simulink model "DvrSimKeybdGD_cs_old"  (R2016a)
settings: Solver=ode5  SolverMode=SingleTasking  StartTime=0.0  StopTime=inf  FixedStep=1/1000  RelTol=1e-3
PreLoadFcn:
  | mbxruntime.callbacks.PreLoadFcn(bdroot);
PostLoadFcn:
  | mbxruntime.callbacks.PostLoadFcn(bdroot);
InitFcn:
  | mbxruntime.callbacks.InitFcn(bdroot);
StartFcn:
  | mbxruntime.callbacks.StartFcn(bdroot);
StopFcn:
  | mbxruntime.callbacks.StopFcn(bdroot);
model workspace (MAT data in the model file):
  mbox_table : struct (value not decoded)
  model_closed = 0
  sim_status = 0
undefined symbols (not defined in the file or in its folder): BMotor1, BMotor2, BrkDelayTime, DControlB, Delay1, Delay2, DiscIntNeverNeededParam, IControlB, JMotor1, JMotor2, PControlB, PreScanCarSimLoadFcn, ratioGearF, ratioGearR, TorqDelayTime, Tstep
undefined symbols (not defined in the file): SteeringColumn, SteeringWheel, WheelL0, WheelL1, WheelR0, WheelR1
libraries: PreScanSimulinkLibrary x35, simulink_extras x26, simulink x26, MyLib x3, Solver_SF x2, pil_lib x1, PreScanUsefulBlocks x1
(part 9 of 12)

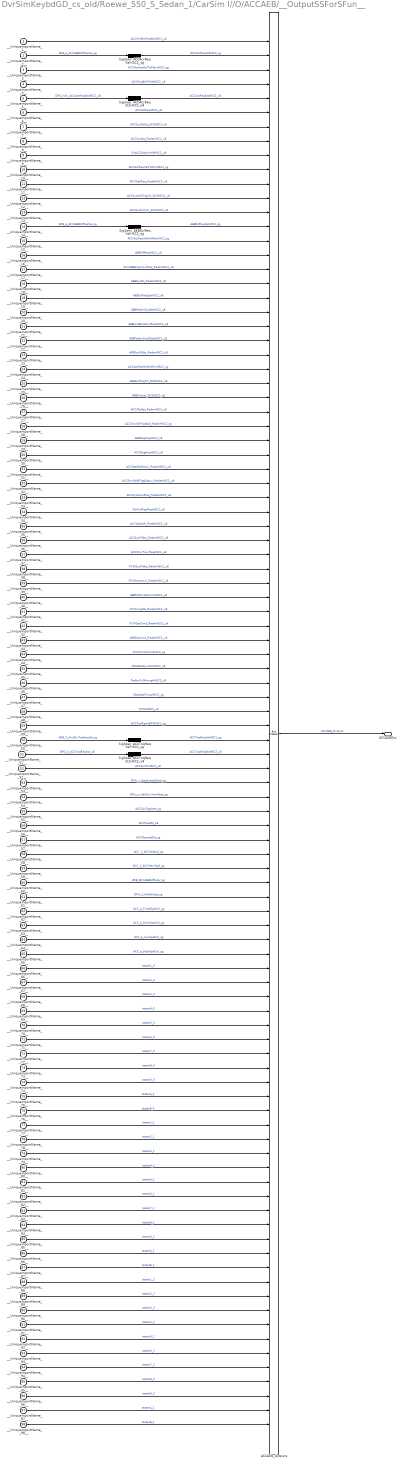
== system DvrSimKeybdGD_cs_old/Roewe_550_S_Sedan_1/CarSim I//O/ACCAEB/__OutputSSForSFun__ ==
  __UniqueInportName__1__ : Inport
  __UniqueInportName__2__ : Inport  Port=2
  __UniqueInportName__3__ : Inport  Port=3
  __UniqueInportName__4__ : Inport  Port=4
  __UniqueInportName__5__ : Inport  Port=5
  __UniqueInportName__6__ : Inport  Port=6
  __UniqueInportName__7__ : Inport  Port=7
  __UniqueInportName__8__ : Inport  Port=8
  __UniqueInportName__9__ : Inport  Port=9
  __UniqueInportName__10__ : Inport  Port=10
  __UniqueInportName__11__ : Inport  Port=11
  __UniqueInportName__12__ : Inport  Port=12
  __UniqueInportName__13__ : Inport  Port=13
  __UniqueInportName__14__ : Inport  Port=14
  __UniqueInportName__15__ : Inport  Port=15
  __UniqueInportName__16__ : Inport  Port=16
  __UniqueInportName__17__ : Inport  Port=17
  __UniqueInportName__18__ : Inport  Port=18
  __UniqueInportName__19__ : Inport  Port=19
  __UniqueInportName__20__ : Inport  Port=20
  __UniqueInportName__21__ : Inport  Port=21
  __UniqueInportName__22__ : Inport  Port=22
  __UniqueInportName__23__ : Inport  Port=23
  __UniqueInportName__24__ : Inport  Port=24
  __UniqueInportName__25__ : Inport  Port=25
  __UniqueInportName__26__ : Inport  Port=26
  __UniqueInportName__27__ : Inport  Port=27
  __UniqueInportName__28__ : Inport  Port=28
  __UniqueInportName__29__ : Inport  Port=29
  __UniqueInportName__30__ : Inport  Port=30
  __UniqueInportName__31__ : Inport  Port=31
  __UniqueInportName__32__ : Inport  Port=32
  __UniqueInportName__33__ : Inport  Port=33
  __UniqueInportName__34__ : Inport  Port=34
  __UniqueInportName__35__ : Inport  Port=35
  __UniqueInportName__36__ : Inport  Port=36
  __UniqueInportName__37__ : Inport  Port=37
  __UniqueInportName__38__ : Inport  Port=38
  __UniqueInportName__39__ : Inport  Port=39
  __UniqueInportName__40__ : Inport  Port=40
  __UniqueInportName__41__ : Inport  Port=41
  __UniqueInportName__42__ : Inport  Port=42
  __UniqueInportName__43__ : Inport  Port=43
  __UniqueInportName__44__ : Inport  Port=44
  __UniqueInportName__45__ : Inport  Port=45
  __UniqueInportName__46__ : Inport  Port=46
  __UniqueInportName__47__ : Inport  Port=47
  __UniqueInportName__48__ : Inport  Port=48
  __UniqueInportName__49__ : Inport  Port=49
  __UniqueInportName__50__ : Inport  Port=50
  __UniqueInportName__51__ : Inport  Port=51
  __UniqueInportName__52__ : Inport  Port=52
  __UniqueInportName__53__ : Inport  Port=53
  __UniqueInportName__54__ : Inport  Port=54
  __UniqueInportName__55__ : Inport  Port=55
  __UniqueInportName__56__ : Inport  Port=56
  __UniqueInportName__57__ : Inport  Port=57
  __UniqueInportName__58__ : Inport  Port=58
  __UniqueInportName__59__ : Inport  Port=59
  __UniqueInportName__60__ : Inport  Port=60
  __UniqueInportName__61__ : Inport  Port=61
  __UniqueInportName__62__ : Inport  Port=62
  __UniqueInportName__63__ : Inport  Port=63
  __UniqueInportName__64__ : Inport  Port=64
  __UniqueInportName__65__ : Inport  Port=65
  __UniqueInportName__66__ : Inport  Port=66
  __UniqueInportName__67__ : Inport  Port=67
  __UniqueInportName__68__ : Inport  Port=68
  __UniqueInportName__69__ : Inport  Port=69
  __UniqueInportName__70__ : Inport  Port=70
  __UniqueInportName__71__ : Inport  Port=71
  __UniqueInportName__72__ : Inport  Port=72
  __UniqueInportName__73__ : Inport  Port=73
  __UniqueInportName__74__ : Inport  Port=74
  __UniqueInportName__75__ : Inport  Port=75
  __UniqueInportName__76__ : Inport  Port=76
  __UniqueInportName__77__ : Inport  Port=77
  __UniqueInportName__78__ : Inport  Port=78
  __UniqueInportName__79__ : Inport  Port=79
  __UniqueInportName__80__ : Inport  Port=80
  __UniqueInportName__81__ : Inport  Port=81
  __UniqueInportName__82__ : Inport  Port=82
  __UniqueInportName__83__ : Inport  Port=83
  __UniqueInportName__84__ : Inport  Port=84
  __UniqueInportName__85__ : Inport  Port=85
  __UniqueInportName__86__ : Inport  Port=86
  __UniqueInportName__87__ : Inport  Port=87
  __UniqueInportName__88__ : Inport  Port=88
  __UniqueInportName__89__ : Inport  Port=89
  __UniqueInportName__90__ : Inport  Port=90
  __UniqueInportName__91__ : Inport  Port=91
  __UniqueInportName__92__ : Inport  Port=92
  __UniqueInportName__93__ : Inport  Port=93
  __UniqueInportName__94__ : Inport  Port=94
  __UniqueInportName__95__ : Inport  Port=95
  __UniqueInportName__96__ : Inport  Port=96
  __UniqueInportName__97__ : Inport  Port=97
  __UniqueInportName__98__ : Inport  Port=98
  ACCAEB_Outputs : BusCreator  Inputs=98
  SigSpec_ACCAccReqStsHSC2_u8 : Demux  Outputs=1
  SigSpec_ACCAccReqValHSC2_sg : Demux  Outputs=1
  SigSpec_ACCToqReqStsHSC2_u8 : Demux  Outputs=1
  SigSpec_ACCToqReqValHSC2_sg : Demux  Outputs=1
  SigSpec_AEBDclReqValHSC2_sg : Demux  Outputs=1
  ACCAEBOut : Outport
  wires:
  __UniqueInportName__2__/1 -> SigSpec_ACCAccReqValHSC2_sg/1  "ARB_a_ACCAEBDclReqVal_sg"
  __UniqueInportName__5__/1 -> SigSpec_ACCAccReqStsHSC2_u8/1  "DPO_indx_ACCAccReqStsHSC2_u8"
  __UniqueInportName__14__/1 -> SigSpec_AEBDclReqValHSC2_sg/1  "ARB_a_ACCAEBDclReqVal_sg"
  __UniqueInportName__50__/1 -> SigSpec_ACCToqReqValHSC2_sg/1  "ARB_T_SmtDrvToqReqVal_sg"
  __UniqueInportName__51__/1 -> SigSpec_ACCToqReqStsHSC2_u8/1  "DPO_is_ACCToqReqSts_u8"
  __UniqueInportName__1__/1 -> ACCAEB_Outputs/1  "ACCMinBrkReqStsHSC2_u8"
  SigSpec_ACCAccReqValHSC2_sg/1 -> ACCAEB_Outputs/2  "ACCAccReqValHSC2_sg"
  __UniqueInportName__3__/1 -> ACCAEB_Outputs/3  "ACCAccReqValTolMaxHSC2_sg"
  __UniqueInportName__4__/1 -> ACCAEB_Outputs/4  "ACCReqBrkPrfrdHSC2_u8"
  SigSpec_ACCAccReqStsHSC2_u8/1 -> ACCAEB_Outputs/5  "ACCAccReqStsHSC2_u8"
  __UniqueInportName__6__/1 -> ACCAEB_Outputs/6  "ACCGoReqHSC2_u8"
  __UniqueInportName__7__/1 -> ACCAEB_Outputs/7  "ACCSysFltSts_SCSHSC2_u8"
  __UniqueInportName__8__/1 -> ACCAEB_Outputs/8  "ACCSysSts_RadarHSC2_u8"
  __UniqueInportName__9__/1 -> ACCAEB_Outputs/9  "ChACCShtdwnMdHSC2_u8"
  __UniqueInportName__10__/1 -> ACCAEB_Outputs/10  "ACCAccReqValTolMinHSC2_sg"
  __UniqueInportName__11__/1 -> ACCAEB_Outputs/11  "ACCSdslReq_RadarHSC2_u8"
  __UniqueInportName__12__/1 -> ACCAEB_Outputs/12  "ACCSysAlvRlngCtr_SCSHSC2_u8"
  __UniqueInportName__13__/1 -> ACCAEB_Outputs/13  "ACCSysChksm_SCSHSC2_u8"
  SigSpec_AEBDclReqValHSC2_sg/1 -> ACCAEB_Outputs/14  "AEBDclReqValHSC2_sg"
  __UniqueInportName__15__/1 -> ACCAEB_Outputs/15  "ACCAccReqValGrdMaxHSC2_sg"
  __UniqueInportName__16__/1 -> ACCAEB_Outputs/16  "AEBPrflReqHSC2_u8"
  __UniqueInportName__17__/1 -> ACCAEB_Outputs/17  "ACCAEBBrkJerkLvlReq_RadarHSC2_u8"
  __UniqueInportName__18__/1 -> ACCAEB_Outputs/18  "AEBSysSts_RadarHSC2_u8"
  __UniqueInportName__19__/1 -> ACCAEB_Outputs/19  "AEBDclReqStsHSC2_u8"
  __UniqueInportName__20__/1 -> ACCAEB_Outputs/20  "AEBPedtrnSysStsHSC2_u8"
  __UniqueInportName__21__/1 -> ACCAEB_Outputs/21  "AEBHydBrkAstLvlReqHSC2_u8"
  __UniqueInportName__22__/1 -> ACCAEB_Outputs/22  "AEBPedtrnSysFltStsHSC2_u8"
  __UniqueInportName__23__/1 -> ACCAEB_Outputs/23  "AEBSysFltSts_RadarHSC2_u8"
  __UniqueInportName__24__/1 -> ACCAEB_Outputs/24  "ACCAccReqValGrdMinHSC2_sg"
  __UniqueInportName__25__/1 -> ACCAEB_Outputs/25  "AEBAlvRlngCtr_SCSHSC2_u8"
  __UniqueInportName__26__/1 -> ACCAEB_Outputs/26  "AEBChksm_SCSHSC2_u8"
  __UniqueInportName__27__/1 -> ACCAEB_Outputs/27  "ACCObjDet_RadarHSC2_u8"
  __UniqueInportName__28__/1 -> ACCAEB_Outputs/28  "ACCDrvrSelTrgtSpd_RadarHSC2_sg"
  __UniqueInportName__29__/1 -> ACCAEB_Outputs/29  "AEBMsgReqHSC2_u8"
  __UniqueInportName__30__/1 -> ACCAEB_Outputs/30  "ACCMsgReqHSC2_u8"
  __UniqueInportName__31__/1 -> ACCAEB_Outputs/31  "ACCDetObjDistLvl_RadarHSC2_u8"
  __UniqueInportName__32__/1 -> ACCAEB_Outputs/32  "ACCDrvrSeldTrgtDistLvl_RadarHSC2_u8"
  __UniqueInportName__33__/1 -> ACCAEB_Outputs/33  "ACCSysCanclReq_RadarHSC2_u8"
  __UniqueInportName__34__/1 -> ACCAEB_Outputs/34  "RdrCalPrgsReqHSC2_u8"
  __UniqueInportName__35__/1 -> ACCAEB_Outputs/35  "ACCGoNotfr_RadarHSC2_u8"
  __UniqueInportName__36__/1 -> ACCAEB_Outputs/36  "ACCSysFltSts_RadarHSC2_u8"
  __UniqueInportName__37__/1 -> ACCAEB_Outputs/37  "ACCDrvrTkovReqHSC2_u8"
  __UniqueInportName__38__/1 -> ACCAEB_Outputs/38  "FCWSysFltSts_RadarHSC2_u8"
  __UniqueInportName__39__/1 -> ACCAEB_Outputs/39  "FCWSnstvtLvl_RadarHSC2_u8"
  __UniqueInportName__40__/1 -> ACCAEB_Outputs/40  "AEBPedtrnDspCmdHSC2_u8"
  __UniqueInportName__41__/1 -> ACCAEB_Outputs/41  "FCWrnngSts_RadarHSC2_u8"
  __UniqueInportName__42__/1 -> ACCAEB_Outputs/42  "FCWDspCmd_RadarHSC2_u8"
  __UniqueInportName__43__/1 -> ACCAEB_Outputs/43  "AEBDspCmd_RadarHSC2_u8"
  __UniqueInportName__44__/1 -> ACCAEB_Outputs/44  "FCWTimeToColHSC2_sg"
  __UniqueInportName__45__/1 -> ACCAEB_Outputs/45  "ObsDataSyncCtrHSC2_u8"
  __UniqueInportName__46__/1 -> ACCAEB_Outputs/46  "PedtrnColWrnngAHSC2_u8"
  __UniqueInportName__47__/1 -> ACCAEB_Outputs/47  "ObsDataTmspHSC2_sg"
  __UniqueInportName__48__/1 -> ACCAEB_Outputs/48  "FCWAHSC2_u8"
  __UniqueInportName__49__/1 -> ACCAEB_Outputs/49  "ACCToqReqValPVHSC2_sg"
  SigSpec_ACCToqReqValHSC2_sg/1 -> ACCAEB_Outputs/50  "ACCToqReqValHSC2_sg"
  SigSpec_ACCToqReqStsHSC2_u8/1 -> ACCAEB_Outputs/51  "ACCToqReqStsHSC2_u8"
  __UniqueInportName__52__/1 -> ACCAEB_Outputs/52  "ACCAlvRCHSC2_u8"
  __UniqueInportName__53__/1 -> ACCAEB_Outputs/53  "DFIn_v_EgoAvgVehSpd_sg"
  __UniqueInportName__54__/1 -> ACCAEB_Outputs/54  "DFIn_yr_VehDynYawRate_sg"
  __UniqueInportName__55__/1 -> ACCAEB_Outputs/55  "ACCSysTgtAccel_sg"
  __UniqueInportName__56__/1 -> ACCAEB_Outputs/56  "ACCReqSts_u8"
  __UniqueInportName__57__/1 -> ACCAEB_Outputs/57  "ACCDesiredDis_sg"
  __UniqueInportName__58__/1 -> ACCAEB_Outputs/58  "ACC_V_ACCSetSpd_sg"
  __UniqueInportName__59__/1 -> ACCAEB_Outputs/59  "ACC_V_ACCMemSpd_sg"
  __UniqueInportName__60__/1 -> ACCAEB_Outputs/60  "ARB_ACCAEBDclReqV_sg"
  __UniqueInportName__61__/1 -> ACCAEB_Outputs/61  "DFIn_V_HdVehSpd_sg"
  __UniqueInportName__62__/1 -> ACCAEB_Outputs/62  "ACC_a_FixedSpdCtrl_sg"
  __UniqueInportName__63__/1 -> ACCAEB_Outputs/63  "ACC_a_EmerSpdCtrl_sg"
  __UniqueInportName__64__/1 -> ACCAEB_Outputs/64  "ACC_a_LowSpdCtrl_sg"
  __UniqueInportName__65__/1 -> ACCAEB_Outputs/65  "ACC_a_HighSpdCtrl_sg"
  __UniqueInportName__66__/1 -> ACCAEB_Outputs/66  "tester1_0"
  __UniqueInportName__67__/1 -> ACCAEB_Outputs/67  "tester2_0"
  __UniqueInportName__68__/1 -> ACCAEB_Outputs/68  "tester3_0"
  __UniqueInportName__69__/1 -> ACCAEB_Outputs/69  "tester4_0"
  __UniqueInportName__70__/1 -> ACCAEB_Outputs/70  "tester5_0"
  __UniqueInportName__71__/1 -> ACCAEB_Outputs/71  "tester6_0"
  __UniqueInportName__72__/1 -> ACCAEB_Outputs/72  "tester7_0"
  __UniqueInportName__73__/1 -> ACCAEB_Outputs/73  "tester8_0"
  __UniqueInportName__74__/1 -> ACCAEB_Outputs/74  "tester9_0"
  __UniqueInportName__75__/1 -> ACCAEB_Outputs/75  "testerA_0"
  __UniqueInportName__76__/1 -> ACCAEB_Outputs/76  "testerB_0"
  __UniqueInportName__77__/1 -> ACCAEB_Outputs/77  "tester1_1"
  __UniqueInportName__78__/1 -> ACCAEB_Outputs/78  "tester2_1"
  __UniqueInportName__79__/1 -> ACCAEB_Outputs/79  "tester3_1"
  __UniqueInportName__80__/1 -> ACCAEB_Outputs/80  "tester4_1"
  __UniqueInportName__81__/1 -> ACCAEB_Outputs/81  "tester5_1"
  __UniqueInportName__82__/1 -> ACCAEB_Outputs/82  "tester6_1"
  __UniqueInportName__83__/1 -> ACCAEB_Outputs/83  "tester7_1"
  __UniqueInportName__84__/1 -> ACCAEB_Outputs/84  "tester8_1"
  __UniqueInportName__85__/1 -> ACCAEB_Outputs/85  "tester9_1"
  __UniqueInportName__86__/1 -> ACCAEB_Outputs/86  "testerA_1"
  __UniqueInportName__87__/1 -> ACCAEB_Outputs/87  "testerB_1"
  __UniqueInportName__88__/1 -> ACCAEB_Outputs/88  "tester1_2"
  __UniqueInportName__89__/1 -> ACCAEB_Outputs/89  "tester2_2"
  __UniqueInportName__90__/1 -> ACCAEB_Outputs/90  "tester3_2"
  __UniqueInportName__91__/1 -> ACCAEB_Outputs/91  "tester4_2"
  __UniqueInportName__92__/1 -> ACCAEB_Outputs/92  "tester5_2"
  __UniqueInportName__93__/1 -> ACCAEB_Outputs/93  "tester6_2"
  __UniqueInportName__94__/1 -> ACCAEB_Outputs/94  "tester7_2"
  __UniqueInportName__95__/1 -> ACCAEB_Outputs/95  "tester8_2"
  __UniqueInportName__96__/1 -> ACCAEB_Outputs/96  "tester9_2"
  __UniqueInportName__97__/1 -> ACCAEB_Outputs/97  "testerA_2"
  __UniqueInportName__98__/1 -> ACCAEB_Outputs/98  "testerB_2"
  ACCAEB_Outputs/1 -> ACCAEBOut/1  "ACCAEB_Outputs"

== system DvrSimKeybdGD_cs_old/Roewe_550_S_Sedan_1/CarSim I//O/ACCAEB In/On Hold ==
  In1 : Inport
  Triggered Subsystem : Subsystem  TreatAsAtomicUnit=on
  Unit Delay : UnitDelay  SampleTime=-1
  Out1 : Outport
  wires:
  Triggered Subsystem/1(Out1) -> Out1/1, Unit Delay/1
  Unit Delay/1 -> Triggered Subsystem/1(In1)
  In1/1 -> Triggered Subsystem/Trigger

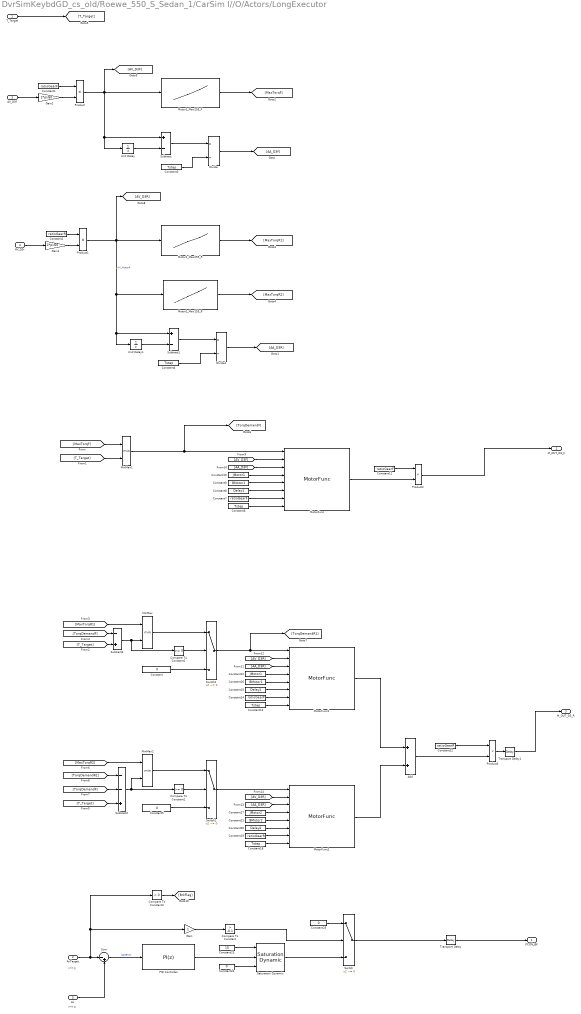
== system DvrSimKeybdGD_cs_old/Roewe_550_S_Sedan_1/CarSim I//O/Actors/LongExecutor ==
  note: unit:g
  note: unit:g
  T_Target : Inport
  AxTarget : Inport  Port=2
  AV_D3f : Inport  Port=3
  AV_D3r : Inport  Port=4
  Ax : Inport  Port=5
  Add : Sum
  Compare To Constant : simulink/Logic and Bit Operations/Compare To Constant  relop=>  const=-0.1  OutDataTypeStr=boolean
  Compare To Constant1 : simulink/Logic and Bit Operations/Compare To Constant  relop=>=  const=0  OutDataTypeStr=boolean
  Compare To Constant2 : simulink/Logic and Bit Operations/Compare To Constant  relop=>=  const=0  OutDataTypeStr=boolean
  Compare To Constant3 : simulink/Logic and Bit Operations/Compare To Constant  relop=<  const=0  OutDataTypeStr=boolean
  Constant{,5,24..25} (4 alike) : Constant  Value=0
  Constant{1,7,11,14} (4 alike) : Constant  Value=ratioGearF
  Constant10 : Constant  Value=JMotor1
  Constant12 : Constant  Value=JMotor1
  Constant{3..4,6,13,18} (5 alike) : Constant  Value=Tstep
  Constant15 : Constant  Value=Delay1
  Constant16 : Constant  Value=BMotor1
  Constant17 : Constant  Value=JMotor2
  Constant19 : Constant  Value=ratioGearR
  Constant2 : Constant  Value=ratioGearR
  Constant20 : Constant  Value=Delay2
  Constant21 : Constant  Value=BMotor2
  Constant22 : Constant  Value=ratioGearR
  Constant23 : Constant  Value=15
  Constant8 : Constant  Value=Delay1
  Constant9 : Constant  Value=BMotor1
  Divide : Product  Inputs=*/
  Divide1 : Product  Inputs=*/
  Gain : Gain
  Gain1 : Gain  Gain=2*pi/60
  Gain2 : Gain  Gain=2*pi/60
  MinMax : MinMax  Inputs=2
  MinMax1 : MinMax  Inputs=2
  MinMax2 : MinMax  Inputs=2
  Motor1_Max255_F : Lookup_n-D  NumberOfTableDimensions=1  BreakpointsForDimension1="[-1047.2,-942.48,-837.76,-733.04,-628.32,-523.6,-418.88,-314.16,-209.44,-104.72,-52.36,-0.1,0,0.1,52.36,104.72,209.44,314.16,418.88,523.6\t628.32,733.04,837.76,942.48,1047.2]"  Table=[-67,-79,-92,-108,-130,-159,-204,-255,-255,-255,-255,-255,255,255,255,255,255,255,204,159,130,108,92,79,67]  InternalRulePriority=Speed  RndMeth=Simplest  InputSameDT=on
  Motor1_Max255_R : Lookup_n-D  NumberOfTableDimensions=1  BreakpointsForDimension1="[-1047.2,-942.48,-837.76,-733.04,-628.32,-523.6,-418.88,-314.16,-209.44,-104.72,-52.36,-0.1,0,0.1,52.36,104.72,209.44,314.16,418.88,523.6\t628.32,733.04,837.76,942.48,1047.2]"  Table=[-67,-79,-92,-108,-130,-159,-204,-255,-255,-255,-255,-255,255,255,255,255,255,255,204,159,130,108,92,79,67]  InternalRulePriority=Speed  RndMeth=Simplest  InputSameDT=on
  Motor2_Max155_R : Lookup_n-D  NumberOfTableDimensions=1  BreakpointsForDimension1="[-1047.2,-942.48,-837.76,-733.04,-628.32,-523.6,-418.88,-314.16,-209.44,-104.72,-52.36,-0.1,0,0.1,52.36,104.72,209.44,314.16,418.88,523.6\t628.32,733.04,837.76,942.48,1047.2]"  Table="[-46.6,-52.3,-58.93,-69,-82.5,-99.5,-124.5,-155,-155,-155\t,-155,-155,155,155,155,155,155,155,124.5,99.5,82.5,69,58.93,52.3,46.6]"  InternalRulePriority=Speed  RndMeth=Simplest  InputSameDT=on
  MotorFunc : MyLib/MotorFunc
  MotorFunc1 : MyLib/MotorFunc
  MotorFunc2 : MyLib/MotorFunc
  PID Controller : simulink/Continuous/PID Controller  Controller=PI  TimeDomain=Discrete-time  SampleTime=0.001  IntegratorMethod=Forward Euler  FilterMethod=Forward Euler  Form=Parallel  UseFilter=on  ControllerParametersSource=internal  P=PControlB  I=IControlB  D=DControlB  N=100  InitialConditionSource=internal  InitialConditionForIntegrator=0  InitialConditionForFilter=0  ExternalReset=none  LimitOutput=off  UpperSaturationLimit=inf  LowerSaturationLimit=-inf  LinearizeAsGain=on  AntiWindupMode=none  Kb=1  TrackingMode=off  Kt=1  PParamMin=[]  PParamMax=[]  IParamMin=[]  IParamMax=[]  DParamMin=[]  DParamMax=[]  NParamMin=[]  NParamMax=[]  KbParamMin=[]  KbParamMax=[]  KtParamMin=[]  KtParamMax=[]  POutMin=[]  POutMax=[]  IOutMin=[]  IOutMax=[]  DOutMin=[]  DOutMax=[]  NOutMin=[]  NOutMax=[]  KbOutMin=[]  KbOutMax=[]  KtOutMin=[]  KtOutMax=[]  IntegratorOutMin=[]  IntegratorOutMax=[]  FilterOutMin=[]  FilterOutMax=[]  SumOutMin=[]  SumOutMax=[]  SumI1OutMin=[]  SumI1OutMax=[]  SumI2OutMin=[]  SumI2OutMax=[]  SumI3OutMin=[]  SumI3OutMax=[]  SumDOutMin=[]  SumDOutMax=[]  SaturationOutMin=[]  SaturationOutMax=[]  IntegratorContinuousStateAttributes=''  IntegratorStateMustResolveToSignalObject=off  IntegratorRTWStateStorageClass=Auto  FilterContinuousStateAttributes=''  FilterStateMustResolveToSignalObject=off  FilterRTWStateStorageClass=Auto  DifferentiatorICPrevScaledInput=0  DifferentiatorOutMin=[]  DifferentiatorOutMax=[]
  Product{,1..3} (4 alike) : Product
  Saturation Dynamic : simulink/Discontinuities/Saturation Dynamic  OutMin=[]  OutMax=[]  OutDataTypeStr=Inherit: Same as second input  OutDataType=fixdt(1, 16)  OutScaling=2^-10  DoSatur=off
  Subtract : Sum  Inputs=+-
  Subtract1 : Sum  Inputs=+-
  Subtract2 : Sum  Inputs=--+
  Subtract3 : Sum  Inputs=-+
  Sum : Sum  Inputs=|-+
  Switch : Switch  Criteria=u2 ~= 0
  Switch1 : Switch  Criteria=u2 ~= 0
  Switch2 : Switch  Criteria=u2 ~= 0
  Transport Delay : TransportDelay  DelayTime=BrkDelayTime
  Transport Delay1 : TransportDelay  DelayTime=TorqDelayTime
  Unit Delay : UnitDelay  SampleTime=-1
  Unit Delay1 : UnitDelay  SampleTime=-1
  PCON_BK : Outport
  M_OUT_D3_F : Outport  Port=2
  M_OUT_D3_R : Outport  Port=3
  wires:
  AV_D3f/1 -> Gain2/1
  Constant1/1 -> Product/1
  AV_D3r/1 -> Gain1/1
  Constant2/1 -> Product1/1
  Product/1 -> [AV_D3F], Unit Delay/1, Subtract/1, Motor1_Max255_F/1
  Unit Delay/1 -> Subtract/2
  Subtract/1 -> Divide/1
  Constant3/1 -> Divide/2
  Motor1_Max255_F/1 -> [MaxTorqF]
  Product1/1 -> [AV_D3R], Unit Delay1/1, Subtract1/1, Motor2_Max155_R/1, Motor1_Max255_R/1  "AV_MotorR"
  Divide/1 -> [AA_D3F]
  Unit Delay1/1 -> Subtract1/2
  Subtract1/1 -> Divide1/1
  Constant4/1 -> Divide1/2
  Divide1/1 -> [AA_D3R]
  Motor1_Max255_R/1 -> [MaxTorqR1]
  Motor2_Max155_R/1 -> [MaxTorqR2]
  T_Target/1 -> [T_Target]
  [MaxTorqF] -> MinMax1/1
  [T_Target] -> MinMax1/2
  MinMax1/1 -> MotorFunc/1, [TorqDemandF]
  [TorqDemandF] -> Subtract3/1
  [T_Target] -> Subtract3/2
  Subtract3/1 -> Compare To Constant2/1, MinMax/2
  [MaxTorqR1] -> MinMax/1
  MinMax/1 -> Switch2/1
  Compare To Constant2/1 -> Switch2/2
  Constant/1 -> Switch2/3
  [TorqDemandF] -> Subtract2/2
  [T_Target] -> Subtract2/3
  Subtract2/1 -> MinMax2/2, Compare To Constant1/1
  [MaxTorqR2] -> MinMax2/1
  MinMax2/1 -> Switch1/1
  Compare To Constant1/1 -> Switch1/2
  Constant5/1 -> Switch1/3
  [TorqDemandR1] -> Subtract2/1
  Constant6/1 -> MotorFunc/8
  Constant7/1 -> MotorFunc/7
  Constant8/1 -> MotorFunc/6
  Constant9/1 -> MotorFunc/5
  Constant10/1 -> MotorFunc/4
  [AV_D3F] -> MotorFunc/2
  [AA_D3F] -> MotorFunc/3
  Constant11/1 -> Product2/1
  Switch2/1 -> MotorFunc1/1, [TorqDemandR1]
  [AV_D3R] -> MotorFunc1/2
  [AA_D3R] -> MotorFunc1/3
  Constant12/1 -> MotorFunc1/4
  Constant16/1 -> MotorFunc1/5
  Constant15/1 -> MotorFunc1/6
  Constant14/1 -> MotorFunc1/7
  Constant13/1 -> MotorFunc1/8
  Switch1/1 -> MotorFunc2/1
  [AV_D3R] -> MotorFunc2/2
  [AA_D3R] -> MotorFunc2/3
  Constant17/1 -> MotorFunc2/4
  Constant21/1 -> MotorFunc2/5
  Constant20/1 -> MotorFunc2/6
  Constant19/1 -> MotorFunc2/7
  Constant18/1 -> MotorFunc2/8
  Constant22/1 -> Product3/1
  Product3/1 -> Transport Delay1/1
  Add/1 -> Product3/2
  MotorFunc1/1 -> Add/1
  MotorFunc2/1 -> Add/2
  Ax/1 -> Sum/2
  Sum/1 -> PID Controller/1  "lastError"
  Constant23/1 -> Saturation Dynamic/1
  Constant24/1 -> Saturation Dynamic/3
  Saturation Dynamic/1 -> Switch/3
  Compare To Constant/1 -> Switch/2
  Constant25/1 -> Switch/1
  Switch/1 -> Transport Delay/1
  Gain1/1 -> Product1/2
  Gain2/1 -> Product/2
  Transport Delay/1 -> PCON_BK/1
  MotorFunc/1 -> Product2/2
  PID Controller/1 -> Saturation Dynamic/2
  AxTarget/1 -> Compare To Constant3/1, Gain/1, Sum/1
  Compare To Constant3/1 -> [BrkFlag]
  Product2/1 -> M_OUT_D3_F/1
  Transport Delay1/1 -> M_OUT_D3_R/1
  Gain/1 -> Compare To Constant/1

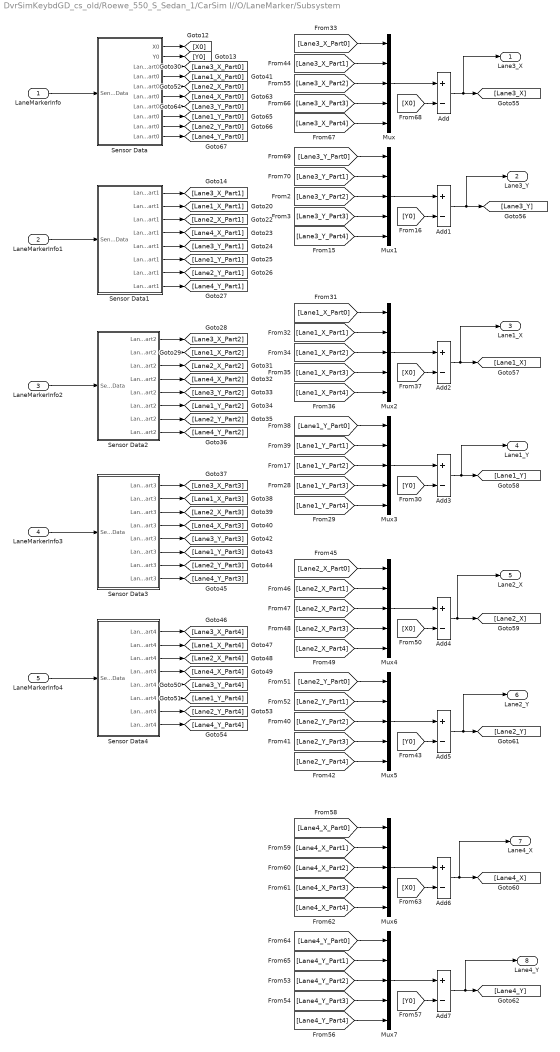
== system DvrSimKeybdGD_cs_old/Roewe_550_S_Sedan_1/CarSim I//O/LaneMarker/Subsystem ==
  LaneMarkerInfo : Inport
  LaneMarkerInfo1 : Inport  Port=2
  LaneMarkerInfo2 : Inport  Port=3
  LaneMarkerInfo3 : Inport  Port=4
  LaneMarkerInfo4 : Inport  Port=5
  Add{,1..7} (8 alike) : Sum  Inputs=+-
  Mux{,1..7} (8 alike) : Mux  Inputs=5
  Sensor Data : Subsystem
  Sensor Data1 : Subsystem
  Sensor Data2 : Subsystem
  Sensor Data3 : Subsystem
  Sensor Data4 : Subsystem
  Lane3_X : Outport
  Lane3_Y : Outport  Port=2
  Lane1_X : Outport  Port=3
  Lane1_Y : Outport  Port=4
  Lane2_X : Outport  Port=5
  Lane2_Y : Outport  Port=6
  Lane4_X : Outport  Port=7
  Lane4_Y : Outport  Port=8
  wires:
  [X0] -> Add4/2
  [Lane4_X_Part2] -> Mux6/3
  [Lane2_Y_Part1] -> Mux5/2
  Mux6/1 -> Add6/1
  [Lane4_X_Part0] -> Mux6/1
  [X0] -> Add6/2
  [Lane4_Y_Part4] -> Mux7/5
  Add/1 -> Lane3_X/1, [Lane3_X]
  [Lane4_Y_Part0] -> Mux7/1
  Add3/1 -> Lane1_Y/1, [Lane1_Y]
  [Lane2_Y_Part0] -> Mux5/1
  Mux5/1 -> Add5/1
  Add6/1 -> Lane4_X/1, [Lane4_X]
  [Lane2_Y_Part3] -> Mux5/4
  Mux7/1 -> Add7/1
  Add4/1 -> Lane2_X/1, [Lane2_X]
  Add1/1 -> Lane3_Y/1, [Lane3_Y]
  [Y0] -> Add5/2
  [Lane4_Y_Part1] -> Mux7/2
  [Lane2_Y_Part2] -> Mux5/3
  [Lane4_Y_Part2] -> Mux7/3
  [Lane4_X_Part3] -> Mux6/4
  [Lane4_X_Part4] -> Mux6/5
  [Y0] -> Add7/2
  [Lane4_X_Part1] -> Mux6/2
  Add7/1 -> Lane4_Y/1, [Lane4_Y]
  Add5/1 -> Lane2_Y/1, [Lane2_Y]
  [Lane4_Y_Part3] -> Mux7/4
  [Lane2_Y_Part4] -> Mux5/5
  Sensor Data4/5(Lane3_Y_Part4) -> [Lane3_Y_Part4]
  Sensor Data2/7(Lane2_Y_Part2) -> [Lane2_Y_Part2]
  Sensor Data3/5(Lane3_Y_Part3) -> [Lane3_Y_Part3]
  [Lane3_X_Part3] -> Mux/4
  Sensor Data2/1(Lane3_X_Part2) -> [Lane3_X_Part2]
  Sensor Data3/1(Lane3_X_Part3) -> [Lane3_X_Part3]
  Sensor Data1/8(Lane4_Y_Part1) -> [Lane4_Y_Part1]
  Sensor Data3/3(Lane2_X_Part3) -> [Lane2_X_Part3]
  Sensor Data4/3(Lane2_X_Part4) -> [Lane2_X_Part4]
  Sensor Data2/6(Lane1_Y_Part2) -> [Lane1_Y_Part2]
  Sensor Data1/6(Lane1_Y_Part1) -> [Lane1_Y_Part1]
  Sensor Data3/2(Lane1_X_Part3) -> [Lane1_X_Part3]
  Sensor Data2/3(Lane2_X_Part2) -> [Lane2_X_Part2]
  Sensor Data3/8(Lane4_Y_Part3) -> [Lane4_Y_Part3]
  Sensor Data4/2(Lane1_X_Part4) -> [Lane1_X_Part4]
  Sensor Data3/7(Lane2_Y_Part3) -> [Lane2_Y_Part3]
  Sensor Data4/7(Lane2_Y_Part4) -> [Lane2_Y_Part4]
  Sensor Data3/6(Lane1_Y_Part3) -> [Lane1_Y_Part3]
  [Lane3_X_Part4] -> Mux/5
  [Lane3_X_Part1] -> Mux/2
  Sensor Data4/4(Lane4_X_Part4) -> [Lane4_X_Part4]
  [X0] -> Add/2
  Sensor Data2/2(Lane1_X_Part2) -> [Lane1_X_Part2]
  Sensor Data1/3(Lane2_X_Part1) -> [Lane2_X_Part1]
  Sensor Data4/6(Lane1_Y_Part4) -> [Lane1_Y_Part4]
  [Lane3_X_Part0] -> Mux/1
  Mux/1 -> Add/1
  [Lane3_Y_Part0] -> Mux1/1
  [Lane3_Y_Part2] -> Mux1/3
  [Lane3_Y_Part4] -> Mux1/5
  [Lane3_Y_Part1] -> Mux1/2
  Mux1/1 -> Add1/1
  [Y0] -> Add1/2
  Sensor Data2/8(Lane4_Y_Part2) -> [Lane4_Y_Part2]
  [Lane1_X_Part4] -> Mux2/5
  [Lane1_Y_Part0] -> Mux3/1
  [Lane1_X_Part3] -> Mux2/4
  [Lane1_Y_Part3] -> Mux3/4
  Sensor Data2/5(Lane3_Y_Part2) -> [Lane3_Y_Part2]
  Sensor Data1/7(Lane2_Y_Part1) -> [Lane2_Y_Part1]
  Sensor Data4/1(Lane3_X_Part4) -> [Lane3_X_Part4]
  Sensor Data4/8(Lane4_Y_Part4) -> [Lane4_Y_Part4]
  Sensor Data3/4(Lane4_X_Part3) -> [Lane4_X_Part3]
  Sensor Data2/4(Lane4_X_Part2) -> [Lane4_X_Part2]
  [Lane3_Y_Part3] -> Mux1/4
  Sensor Data1/5(Lane3_Y_Part1) -> [Lane3_Y_Part1]
  [Lane1_X_Part1] -> Mux2/2
  [Lane1_X_Part2] -> Mux2/3
  Mux2/1 -> Add2/1
  [X0] -> Add2/2
  [Lane1_X_Part0] -> Mux2/1
  [Lane1_Y_Part2] -> Mux3/3
  [Lane1_Y_Part4] -> Mux3/5
  [Lane3_X_Part2] -> Mux/3
  [Y0] -> Add3/2
  [Lane2_X_Part0] -> Mux4/1
  [Lane2_X_Part2] -> Mux4/3
  [Lane1_Y_Part1] -> Mux3/2
  Mux3/1 -> Add3/1
  Mux4/1 -> Add4/1
  [Lane2_X_Part3] -> Mux4/4
  [Lane2_X_Part1] -> Mux4/2
  [Lane2_X_Part4] -> Mux4/5
  Sensor Data/2(Y0) -> [Y0]
  Sensor Data/3(Lane3_X_Part0) -> [Lane3_X_Part0]
  Sensor Data/6(Lane4_X_Part0) -> [Lane4_X_Part0]
  Sensor Data/7(Lane3_Y_Part0) -> [Lane3_Y_Part0]
  Sensor Data/1(X0) -> [X0]
  Sensor Data/4(Lane1_X_Part0) -> [Lane1_X_Part0]
  Sensor Data/8(Lane1_Y_Part0) -> [Lane1_Y_Part0]
  Sensor Data/9(Lane2_Y_Part0) -> [Lane2_Y_Part0]
  Sensor Data/10(Lane4_Y_Part0) -> [Lane4_Y_Part0]
  Sensor Data1/1(Lane3_X_Part1) -> [Lane3_X_Part1]
  Sensor Data/5(Lane2_X_Part0) -> [Lane2_X_Part0]
  Sensor Data1/2(Lane1_X_Part1) -> [Lane1_X_Part1]
  Sensor Data1/4(Lane4_X_Part1) -> [Lane4_X_Part1]
  Add2/1 -> Lane1_X/1, [Lane1_X]
  LaneMarkerInfo/1 -> Sensor Data/1(Sensor Data)
  LaneMarkerInfo1/1 -> Sensor Data1/1(Sensor Data)
  LaneMarkerInfo2/1 -> Sensor Data2/1(Sensor Data)
  LaneMarkerInfo3/1 -> Sensor Data3/1(Sensor Data)
  LaneMarkerInfo4/1 -> Sensor Data4/1(Sensor Data)

== system DvrSimKeybdGD_cs_old/Roewe_550_S_Sedan_1/CarSim_Vehicle/CarSim2PreScanSTATE/Transformation_SprungMassCarSim2PreScan ==
  In1 : Inport
  Demux : Demux  Outputs=3
  Ini z-position VEHICLE wrt GLOBAL axis system [m] : Constant  Value=z0
  Mux : Mux  Inputs=3
  Sum1 : Sum  Inputs=+-
  Out1 : Outport
  wires:
  Mux/1 -> Out1/1
  Ini z-position VEHICLE wrt GLOBAL axis system [m]/1 -> Sum1/2
  Demux/1 -> Mux/1
  Sum1/1 -> Mux/3
  Demux/3 -> Sum1/1
  Demux/2 -> Mux/2
  In1/1 -> Demux/1

== system DvrSimKeybdGD_cs_old/Roewe_550_S_Sedan_1/CarSim_Vehicle/CarSim2PreScan_BUS/Steering ==
  SteeringWheel_In : Inport
  AvoidDivisionByZero : Subsystem
  Bus Creator4 : BusCreator  Inputs=1
  DefaultValue : Constant  Value=16
  Demux2 : Demux  Outputs=2
  Divide : Product  Inputs=*/
  Switch : Switch  Criteria=u2 ~= 0
  Steering : Outport
  wires:
  AvoidDivisionByZero/1(Out1) -> Divide/2
  Switch/1 -> Bus Creator4/1  "SteeringRatio_[-]"
  DefaultValue/1 -> Switch/3
  Divide/1 -> Switch/1, Switch/2  "Steering_Ration[-]"
  Demux2/2 -> AvoidDivisionByZero/1(In1)  "Axle1ReducedSW"
  Demux2/1 -> Divide/1  "SteeringWheelAngle_[deg]"
  Bus Creator4/1 -> Steering/1  "Steering"
  SteeringWheel_In/1 -> Demux2/1

== system DvrSimKeybdGD_cs_old/Roewe_550_S_Sedan_1/CarSim_Vehicle/CarSim2PreScan_BUS/Vehicle ==
  v_VehicleCoG[x;y;z][km|h] : Inport
  Bus Creator1 : BusCreator  Inputs=1
  Bus Creator7 : BusCreator  Inputs=1
  Bus Creator8 : BusCreator  Inputs=3
  Demux : Demux  Outputs=3
  Vehicle : Outport
  wires:
  Demux/3 -> Bus Creator8/3  "v_Vehicle[z][km|h]"
  Demux/2 -> Bus Creator8/2  "v_Vehicle[y][km|h]"
  Demux/1 -> Bus Creator8/1  "v_Vehicle[x][km|h]"
  Bus Creator7/1 -> Bus Creator1/1  "Velocities"
  Bus Creator8/1 -> Bus Creator7/1  "Linear"
  Bus Creator1/1 -> Vehicle/1  "Vehicle"
  v_VehicleCoG[x;y;z][km|h]/1 -> Demux/1

== system DvrSimKeybdGD_cs_old/Roewe_550_S_Sedan_1/CarSim_Vehicle/CarSim2PreScan_BUS/Wheel ==
  SprungMass_Pos_Global[x;y;z][m] : Inport
  SprungMass_Angle_Global[x;y;z][deg] : Inport  Port=2
  CarSim_Pos_Wheel_[FL;FR;RL;RR][x;y;z][m] : Inport  Port=3
  CarSim_Angle_Wheel_[FL;FR;RL;RR][x;y;z][deg;rev;deg] : Inport  Port=4
  Bus Creator3 : BusCreator  Inputs=2
  Bus Creator6 : BusCreator  Inputs=1
  Convert CarSim to PreScan Wheel Position : Subsystem
  Convert CarSim to PreScan Wheel Rotation : Subsystem
  Demux : Demux  Outputs=[3 3 3 3]
  Demux1 : Demux  Outputs=[3 3 3 3]
  Wheel : Outport
  wires:
  SprungMass_Angle_Global[x;y;z][deg]/1 -> Convert CarSim to PreScan Wheel Rotation/5(Angle_Vehicle[x;y;z][deg]), Convert CarSim to PreScan Wheel Position/2(SprungMass_Angle_Global[x;y;z][deg])
  SprungMass_Pos_Global[x;y;z][m]/1 -> Convert CarSim to PreScan Wheel Position/1(SprungMass_Pos_Global[x;y;z][m])
  CarSim_Angle_Wheel_[FL;FR;RL;RR][x;y;z][deg;rev;deg]/1 -> Demux1/1
  Demux1/4 -> Convert CarSim to PreScan Wheel Rotation/4(CarSim_Angle_RR_Wheel_CoorSys_V[deg;rev;deg])  "CarSim_Angle_RR_Wheel_CoorSys_V[deg;rev;deg]"
  Demux1/3 -> Convert CarSim to PreScan Wheel Rotation/3(CarSim_Angle_RL_Wheel_CoorSys_V[deg;rev;deg])  "CarSim_Angle_RL_Wheel_CoorSys_V[deg;rev;deg]"
  Demux1/2 -> Convert CarSim to PreScan Wheel Rotation/2(CarSim_Angle_FR_Wheel_CoorSys_V[deg;rev;deg])  "CarSim_Angle_FR_Wheel_CoorSys_V[deg;rev;deg]"
  Demux1/1 -> Convert CarSim to PreScan Wheel Rotation/1(CarSim_Angle_FL_Wheel_CoorSys_V[deg;rev;deg])  "CarSim_Angle_FL_Wheel_CoorSys_V[deg;rev;deg]"
  CarSim_Pos_Wheel_[FL;FR;RL;RR][x;y;z][m]/1 -> Demux/1
  Demux/4 -> Convert CarSim to PreScan Wheel Position/6(CarSim_Pos_RR_Wheel[x;y;z][m])  "CarSim_Pos_RR_Wheel[x;y;z][m]"
  Demux/3 -> Convert CarSim to PreScan Wheel Position/5(CarSim_Pos_RL_Wheel[x;y;z][m])  "CarSim_Pos_RL_Wheel[x;y;z][m]"
  Demux/2 -> Convert CarSim to PreScan Wheel Position/4(CarSim_Pos_FR_Wheel[x;y;z][m])  "CarSim_Pos_FR_Wheel[x;y;z][m]"
  Demux/1 -> Convert CarSim to PreScan Wheel Position/3(CarSim_Pos_FL_Wheel[x;y;z][m])  "CarSim_Pos_FL_Wheel[x;y;z][m]"
  Bus Creator6/1 -> Wheel/1  "Wheel"
  Bus Creator3/1 -> Bus Creator6/1  "Position"
  Convert CarSim to PreScan Wheel Rotation/1(PreScanWheel_Rot) -> Bus Creator3/2
  Convert CarSim to PreScan Wheel Position/1(PreScanWheel_Pos) -> Bus Creator3/1

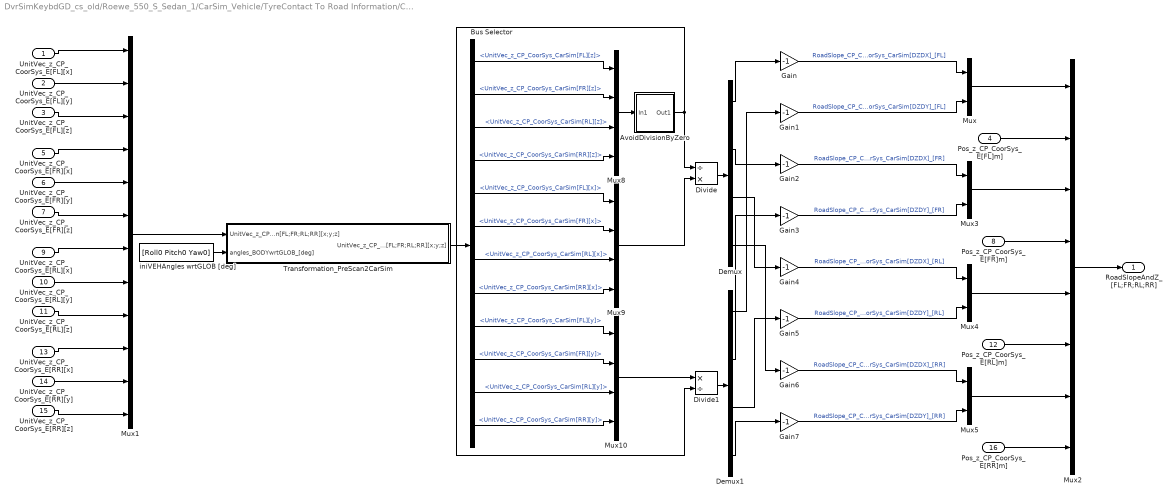
== system DvrSimKeybdGD_cs_old/Roewe_550_S_Sedan_1/CarSim_Vehicle/TyreContact To Road Information/Contact To Road Information ==
  UnitVec_z_CP_CoorSys_E[FL][x] : Inport
  UnitVec_z_CP_CoorSys_E[FL][y] : Inport  Port=2
  UnitVec_z_CP_CoorSys_E[FL][z] : Inport  Port=3
  " Pos_z_CP_CoorSys_E[FL]m]" : Inport  Port=4
  UnitVec_z_CP_CoorSys_E[FR][x] : Inport  Port=5
  UnitVec_z_CP_CoorSys_E[FR][y] : Inport  Port=6
  UnitVec_z_CP_CoorSys_E[FR][z] : Inport  Port=7
  " Pos_z_CP_CoorSys_E[FR]m]" : Inport  Port=8
  UnitVec_z_CP_CoorSys_E[RL][x] : Inport  Port=9
  UnitVec_z_CP_CoorSys_E[RL][y] : Inport  Port=10
  UnitVec_z_CP_CoorSys_E[RL][z] : Inport  Port=11
  " Pos_z_CP_CoorSys_E[RL]m]" : Inport  Port=12
  UnitVec_z_CP_CoorSys_E[RR][x] : Inport  Port=13
  UnitVec_z_CP_CoorSys_E[RR][y] : Inport  Port=14
  UnitVec_z_CP_CoorSys_E[RR][z] : Inport  Port=15
  " Pos_z_CP_CoorSys_E[RR]m]" : Inport  Port=16
  AvoidDivisionByZero : Subsystem
  Bus Selector : BusSelector  OutputSignals=UnitVec_z_CP_CoorSys_CarSim[FL][x;y;z].UnitVec_z_CP_CoorSys_CarSim[FL][z],UnitVec_z_CP_CoorSys_CarSim[FR][x;y;z].UnitVec_z_CP_CoorSys_CarSim[FR][z],UnitVec_z_CP_CoorSys_CarSim[RL][x;y;z].UnitVec_z_CP_CoorSys_CarSim[RL][z],UnitVec_z_CP_CoorSys_CarSim[RR][x;y;z].UnitVec_z_CP_CoorSys_CarSim[RR][z],UnitVec_z_CP_CoorSys_CarSim[FL][x;y;z].UnitVec_z_CP_CoorSys_CarSim[FL][x],UnitVec_z_CP_CoorSys_CarSim[FR][x;y;z].UnitVec_z_CP_CoorSys_CarSim[FR][x],UnitVec_z_CP_CoorSys_CarSim[RL][x;y;z].UnitVec_z_CP_CoorSys_CarSim[RL][x],UnitVec_z_CP_CoorSys_CarSim[RR][x;y;z].UnitVec_z_CP_CoorSys_CarSim[RR][x],UnitVec_z_CP_CoorSys_CarSim[FL][x;y;z].UnitVec_z_CP_CoorSys_CarSim[FL][y],UnitVec_z_CP_CoorSys_CarSim[FR][x;y;z].UnitVec_z_CP_CoorSys_CarSim[FR][y],UnitVec_z_CP_CoorSys_CarSim[RL][x;y;z].UnitVec_z_CP_CoorSys_CarSim[RL][y],UnitVec_z_CP_CoorSys_CarSim[RR][x;y;z].UnitVec_z_CP_CoorSys_CarSim[RR][y]
  Demux : Demux
  Demux1 : Demux
  Divide : Product  Inputs=/*
  Divide1 : Product  Inputs=*/
  Gain{,1..7} (8 alike) : Gain  Gain=-1
  Mux{,3..5} (4 alike) : Mux  Inputs=2
  Mux1 : Mux  Inputs=12
  Mux10 : Mux
  Mux2 : Mux  Inputs=[2 1 2 1 2 1 2 1]
  Mux8 : Mux
  Mux9 : Mux
  Transformation_PreScan2CarSim : Subsystem
  iniVEHAngles wrtGLOB [deg] : Constant  Value=[Roll0 Pitch0 Yaw0]
  RoadSlopeAndZ_[FL;FR;RL;RR] : Outport
  wires:
  AvoidDivisionByZero/1(Out1) -> Divide1/2, Divide/1
  Demux1/4 -> Gain7/1
  Demux/4 -> Gain6/1
  Demux1/3 -> Gain5/1
  Demux/3 -> Gain4/1
  Demux1/2 -> Gain3/1
  Demux/2 -> Gain2/1
  Demux/1 -> Gain/1
  Demux1/1 -> Gain1/1
  Divide1/1 -> Demux1/1
  Divide/1 -> Demux/1
  Mux10/1 -> Divide1/1
  Mux9/1 -> Divide/2
  Mux8/1 -> AvoidDivisionByZero/1(In1)
  Bus Selector/12 -> Mux10/4  "<UnitVec_z_CP_CoorSys_CarSim[RR][y]>"
  Bus Selector/11 -> Mux10/3  "<UnitVec_z_CP_CoorSys_CarSim[RL][y]>"
  Bus Selector/10 -> Mux10/2  "<UnitVec_z_CP_CoorSys_CarSim[FR][y]>"
  Bus Selector/9 -> Mux10/1  "<UnitVec_z_CP_CoorSys_CarSim[FL][y]>"
  Bus Selector/8 -> Mux9/4  "<UnitVec_z_CP_CoorSys_CarSim[RR][x]>"
  Bus Selector/7 -> Mux9/3  "<UnitVec_z_CP_CoorSys_CarSim[RL][x]>"
  Bus Selector/6 -> Mux9/2  "<UnitVec_z_CP_CoorSys_CarSim[FR][x]>"
  Bus Selector/5 -> Mux9/1  "<UnitVec_z_CP_CoorSys_CarSim[FL][x]>"
  Bus Selector/4 -> Mux8/4  "<UnitVec_z_CP_CoorSys_CarSim[RR][z]>"
  Bus Selector/3 -> Mux8/3  "<UnitVec_z_CP_CoorSys_CarSim[RL][z]>"
  Bus Selector/2 -> Mux8/2  "<UnitVec_z_CP_CoorSys_CarSim[FR][z]>"
  Bus Selector/1 -> Mux8/1  "<UnitVec_z_CP_CoorSys_CarSim[FL][z]>"
  Mux5/1 -> Mux2/7
  Mux4/1 -> Mux2/5
  Mux3/1 -> Mux2/3
  " Pos_z_CP_CoorSys_E[FL]m]"/1 -> Mux2/2
  Mux/1 -> Mux2/1
  Gain/1 -> Mux/1  "RoadSlope_CP_CoorSys_CarSim[DZDX]_[FL]"
  " Pos_z_CP_CoorSys_E[RR]m]"/1 -> Mux2/8
  " Pos_z_CP_CoorSys_E[RL]m]"/1 -> Mux2/6
  " Pos_z_CP_CoorSys_E[FR]m]"/1 -> Mux2/4
  Transformation_PreScan2CarSim/1(UnitVec_z_CP_CoorSys _CarSim[FL;FR;RL;RR][x;y;z]) -> Bus Selector/1
  UnitVec_z_CP_CoorSys_E[RR][z]/1 -> Mux1/12
  UnitVec_z_CP_CoorSys_E[RR][y]/1 -> Mux1/11
  UnitVec_z_CP_CoorSys_E[RR][x]/1 -> Mux1/10
  UnitVec_z_CP_CoorSys_E[RL][z]/1 -> Mux1/9
  UnitVec_z_CP_CoorSys_E[RL][y]/1 -> Mux1/8
  UnitVec_z_CP_CoorSys_E[RL][x]/1 -> Mux1/7
  UnitVec_z_CP_CoorSys_E[FR][z]/1 -> Mux1/6
  UnitVec_z_CP_CoorSys_E[FR][y]/1 -> Mux1/5
  UnitVec_z_CP_CoorSys_E[FR][x]/1 -> Mux1/4
  UnitVec_z_CP_CoorSys_E[FL][z]/1 -> Mux1/3
  UnitVec_z_CP_CoorSys_E[FL][y]/1 -> Mux1/2
  UnitVec_z_CP_CoorSys_E[FL][x]/1 -> Mux1/1
  Mux1/1 -> Transformation_PreScan2CarSim/1(UnitVec_z_CP_CoorSys_PreScan[FL;FR;RL;RR][x;y;z])
  iniVEHAngles wrtGLOB [deg]/1 -> Transformation_PreScan2CarSim/2(angles_BODYwrtGLOB_[deg])
  Mux2/1 -> RoadSlopeAndZ_[FL;FR;RL;RR]/1
  Gain1/1 -> Mux/2  "RoadSlope_CP_CoorSys_CarSim[DZDY]_[FL]"
  Gain2/1 -> Mux3/1  "RoadSlope_CP_CoorSys_CarSim[DZDX]_[FR]"
  Gain3/1 -> Mux3/2  "RoadSlope_CP_CoorSys_CarSim[DZDY]_[FR]"
  Gain4/1 -> Mux4/1  "RoadSlope_CP_CoorSys_CarSim[DZDX]_[RL]"
  Gain5/1 -> Mux4/2  "RoadSlope_CP_CoorSys_CarSim[DZDY]_[RL]"
  Gain6/1 -> Mux5/1  "RoadSlope_CP_CoorSys_CarSim[DZDX]_[RR]"
  Gain7/1 -> Mux5/2  "RoadSlope_CP_CoorSys_CarSim[DZDY]_[RR]"

== system DvrSimKeybdGD_cs_old/Roewe_550_S_Sedan_1/PreScan_RayCast_Contact_Sensor/Vehicle Local to World/state2FullState ==
  note: AnglesBODY
      | wrtVEH
  note: AnglesVEHICLE
      | wrtGLOB
  note: AnglesBODY
      | wrt GLOB
  note: mode: Dynamics
      | VelVEHICLE
      | wrt VEH
  note: mode: Positioning
      | VelVEHICLE
      | wrt INI
  note: Angles
      | wrtINI
  note: wrt GLOB
  dx,dy,dz [m/s] R,P,Y [rad] : Inport
  ini VEHpos wrt GLOB axis system [m] : Inport  Port=2
  iniBODY Angles wrt VEH axis system [deg] : Inport  Port=3
  iniVEH Angles wrt GLOB axis system [deg] : Inport  Port=4
  Degrees to Radians : simulink_extras/Transformations/Degrees to Radians
  Degrees to Radians1 : simulink_extras/Transformations/Degrees to Radians
  Demux1 : Demux  Outputs=[3 3 3]
  Demux2 : Demux  Outputs=[2 1]
  Demux3 : Demux  Outputs=2
  Mux : Mux  Inputs=[3 3]
  Sum : Sum  Inputs=|++
  Sum1 : Sum
  Sum2 : Sum
  Sum3 : Sum
  Terminator : Terminator
  Transformation_BODY2GLOBAL1 : Subsystem
  limit roll : Subsystem
  mux2 : Mux  Inputs=3
  mux3 : Mux  Inputs=3
  pitch_vehicle : Constant  Value=0
  roll_vehicle : Constant  Value=0
  yaw_body : Constant  Value=0
  State : Outport
  wires:
  Demux1/2 -> Terminator/1
  limit roll/1(RPYcor) -> Mux/2  "AnglesBODY wrt  GLOB"
  Mux/1 -> State/1
  iniVEH Angles wrt GLOB axis system [deg]/1 -> Degrees to Radians/1
  iniBODY Angles wrt VEH axis system [deg]/1 -> Degrees to Radians1/1
  Sum/1 -> limit roll/1(RPY)
  roll_vehicle/1 -> mux3/1  "roll"
  pitch_vehicle/1 -> mux3/2  "pitch"
  mux2/1 -> Sum1/1
  yaw_body/1 -> mux2/3  "yaw"
  mux3/1 -> Sum2/1
  Sum2/1 -> Sum/2
  dx,dy,dz [m/s] R,P,Y [rad]/1 -> Demux1/1
  Demux1/1 -> Transformation_BODY2GLOBAL1/1(POSvector_BODY_[m])
  Sum1/1 -> Sum/1
  Transformation_BODY2GLOBAL1/1(POSvector_GLOBAL_[m]) -> Sum3/1
  Sum3/1 -> Mux/1  "PosVEH wrt  GLOB"
  Demux2/2 -> mux3/3  "yaw"
  Demux2/1 -> Demux3/1
  Demux1/3 -> Demux2/1
  Demux3/1 -> mux2/1  "roll"
  Degrees to Radians1/1 -> Sum1/2
  Degrees to Radians/1 -> Transformation_BODY2GLOBAL1/2(angles_BODYwrtGLOB_[rad]), Sum2/2
  ini VEHpos wrt GLOB axis system [m]/1 -> Sum3/2
  Demux3/2 -> mux2/2  "pitch"

== system DvrSimKeybdGD_cs_old/Roewe_550_S_Sedan_1/PreScan_RayCast_Contact_Sensor/Wheels = 4/wheelposeFL ==
  vector : Inport  OutDataTypeStr=double  PortDimensions=7
  Bus Creator : BusCreator  Inputs='POSITION','ORIENTATION'  OutDataTypeStr=Bus: PRESCAN_POSEA_DATA  NonVirtualBus=on
  Bus Creator1 : BusCreator  Inputs='X','Y','Z'  OutDataTypeStr=Bus: PRESCAN_XYZ_DATA  NonVirtualBus=on
  Bus Creator3 : BusCreator  Inputs='X','Y','Z','Angle'  OutDataTypeStr=Bus: PRESCAN_AXISANGLE_DATA  NonVirtualBus=on
  Demux : Demux  Outputs=7
  bus : Outport  OutDataTypeStr=Bus: PRESCAN_POSEA_DATA
  wires:
  Bus Creator1/1 -> Bus Creator/1  "POSITION"
  Bus Creator3/1 -> Bus Creator/2  "ORIENTATION"
  Bus Creator/1 -> bus/1
  Demux/1 -> Bus Creator1/1  "X"
  Demux/2 -> Bus Creator1/2  "Y"
  Demux/3 -> Bus Creator1/3  "Z"
  Demux/4 -> Bus Creator3/1  "X"
  Demux/5 -> Bus Creator3/2  "Y"
  Demux/6 -> Bus Creator3/3  "Z"
  Demux/7 -> Bus Creator3/4  "Angle"
  vector/1 -> Demux/1

== system DvrSimKeybdGD_cs_old/Roewe_550_S_Sedan_1/PreScan_RayCast_Contact_Sensor/Wheels = 4/wheelposeFR ==
  vector : Inport  OutDataTypeStr=double  PortDimensions=7
  Bus Creator : BusCreator  Inputs='POSITION','ORIENTATION'  OutDataTypeStr=Bus: PRESCAN_POSEA_DATA  NonVirtualBus=on
  Bus Creator1 : BusCreator  Inputs='X','Y','Z'  OutDataTypeStr=Bus: PRESCAN_XYZ_DATA  NonVirtualBus=on
  Bus Creator3 : BusCreator  Inputs='X','Y','Z','Angle'  OutDataTypeStr=Bus: PRESCAN_AXISANGLE_DATA  NonVirtualBus=on
  Demux : Demux  Outputs=7
  bus : Outport  OutDataTypeStr=Bus: PRESCAN_POSEA_DATA
  wires:
  Bus Creator1/1 -> Bus Creator/1  "POSITION"
  Bus Creator3/1 -> Bus Creator/2  "ORIENTATION"
  Bus Creator/1 -> bus/1
  Demux/1 -> Bus Creator1/1  "X"
  Demux/2 -> Bus Creator1/2  "Y"
  Demux/3 -> Bus Creator1/3  "Z"
  Demux/4 -> Bus Creator3/1  "X"
  Demux/5 -> Bus Creator3/2  "Y"
  Demux/6 -> Bus Creator3/3  "Z"
  Demux/7 -> Bus Creator3/4  "Angle"
  vector/1 -> Demux/1

== system DvrSimKeybdGD_cs_old/Roewe_550_S_Sedan_1/PreScan_RayCast_Contact_Sensor/Wheels = 4/wheelposeRL ==
  vector : Inport  OutDataTypeStr=double  PortDimensions=7
  Bus Creator : BusCreator  Inputs='POSITION','ORIENTATION'  OutDataTypeStr=Bus: PRESCAN_POSEA_DATA  NonVirtualBus=on
  Bus Creator1 : BusCreator  Inputs='X','Y','Z'  OutDataTypeStr=Bus: PRESCAN_XYZ_DATA  NonVirtualBus=on
  Bus Creator3 : BusCreator  Inputs='X','Y','Z','Angle'  OutDataTypeStr=Bus: PRESCAN_AXISANGLE_DATA  NonVirtualBus=on
  Demux : Demux  Outputs=7
  bus : Outport  OutDataTypeStr=Bus: PRESCAN_POSEA_DATA
  wires:
  Bus Creator1/1 -> Bus Creator/1  "POSITION"
  Bus Creator3/1 -> Bus Creator/2  "ORIENTATION"
  Bus Creator/1 -> bus/1
  Demux/1 -> Bus Creator1/1  "X"
  Demux/2 -> Bus Creator1/2  "Y"
  Demux/3 -> Bus Creator1/3  "Z"
  Demux/4 -> Bus Creator3/1  "X"
  Demux/5 -> Bus Creator3/2  "Y"
  Demux/6 -> Bus Creator3/3  "Z"
  Demux/7 -> Bus Creator3/4  "Angle"
  vector/1 -> Demux/1

== system DvrSimKeybdGD_cs_old/Roewe_550_S_Sedan_1/PreScan_RayCast_Contact_Sensor/Wheels = 4/wheelposeRR ==
  vector : Inport  OutDataTypeStr=double  PortDimensions=7
  Bus Creator : BusCreator  Inputs='POSITION','ORIENTATION'  OutDataTypeStr=Bus: PRESCAN_POSEA_DATA  NonVirtualBus=on
  Bus Creator1 : BusCreator  Inputs='X','Y','Z'  OutDataTypeStr=Bus: PRESCAN_XYZ_DATA  NonVirtualBus=on
  Bus Creator3 : BusCreator  Inputs='X','Y','Z','Angle'  OutDataTypeStr=Bus: PRESCAN_AXISANGLE_DATA  NonVirtualBus=on
  Demux : Demux  Outputs=7
  bus : Outport  OutDataTypeStr=Bus: PRESCAN_POSEA_DATA
  wires:
  Bus Creator1/1 -> Bus Creator/1  "POSITION"
  Bus Creator3/1 -> Bus Creator/2  "ORIENTATION"
  Bus Creator/1 -> bus/1
  Demux/1 -> Bus Creator1/1  "X"
  Demux/2 -> Bus Creator1/2  "Y"
  Demux/3 -> Bus Creator1/3  "Z"
  Demux/4 -> Bus Creator3/1  "X"
  Demux/5 -> Bus Creator3/2  "Y"
  Demux/6 -> Bus Creator3/3  "Z"
  Demux/7 -> Bus Creator3/4  "Angle"
  vector/1 -> Demux/1

== system DvrSimKeybdGD_cs_old/Roewe_550_S_Sedan_1/PreScan_RayCast_Contact_Sensor/Wheels Local to World/conv_RotWheelFL ==
  BryantISO [deg] : Inport
  Fcn10 : Fcn  Expr=cos(u(1))*sin(u(3))+sin(u(1))*sin(u(2))*cos(u(3))
  Fcn11 : Fcn  Expr=sin(u(1))*sin(u(3))-cos(u(1))*sin(u(2))*cos(u(3))
  Fcn12 : Fcn  Expr=-cos(u(2))*sin(u(3))
  Fcn13 : Fcn  Expr=cos(u(1))*cos(u(3))-sin(u(1))*sin(u(2))*sin(u(3))
  Fcn14 : Fcn  Expr=sin(u(1))*cos(u(3))+cos(u(1))*sin(u(2))*sin(u(3))
  Fcn15 : Fcn  Expr=sin(u(2))
  Fcn16 : Fcn  Expr=-sin(u(1))*cos(u(2))
  Fcn17 : Fcn  Expr=cos(u(1))*cos(u(2))
  Fcn9 : Fcn  Expr=cos(u(2))*cos(u(3))
  Mux1 : Mux  Inputs=9
  RotMat2AxisAngle : Subsystem
  deg2rad : Gain  Gain=pi/180
  xyz 2 zxy : Selector  InputPortWidth=3  IndexOptions=Index vector (dialog)  Indices=[3 1 2]  OutputSizes=1
  zxy 2 xyz : Selector  InputPortWidth=4  IndexOptions=Index vector (dialog)  Indices=[2 3 1 4]  OutputSizes=1
  QuaternionVisu [rad] : Outport
  wires:
  Fcn9/1 -> Mux1/1
  Fcn10/1 -> Mux1/2
  Fcn11/1 -> Mux1/3
  Fcn12/1 -> Mux1/4
  Fcn13/1 -> Mux1/5
  Fcn14/1 -> Mux1/6
  Fcn15/1 -> Mux1/7
  Fcn16/1 -> Mux1/8
  Fcn17/1 -> Mux1/9
  Mux1/1 -> RotMat2AxisAngle/1(RotMat_Visu)  "RotationMatrix Visu"
  RotMat2AxisAngle/1(Angles_Visu) -> zxy 2 xyz/1
  BryantISO [deg]/1 -> xyz 2 zxy/1  "BryantAngles rotx roty rotz Visu"
  deg2rad/1 -> Fcn9/1, Fcn10/1, Fcn11/1, Fcn12/1, Fcn13/1, Fcn14/1, Fcn15/1, Fcn16/1, Fcn17/1
  xyz 2 zxy/1 -> deg2rad/1
  zxy 2 xyz/1 -> QuaternionVisu [rad]/1

== system DvrSimKeybdGD_cs_old/Roewe_550_S_Sedan_1/PreScan_RayCast_Contact_Sensor/Wheels Local to World/conv_RotWheelFR ==
  BryantISO [deg] : Inport
  Fcn10 : Fcn  Expr=cos(u(1))*sin(u(3))+sin(u(1))*sin(u(2))*cos(u(3))
  Fcn11 : Fcn  Expr=sin(u(1))*sin(u(3))-cos(u(1))*sin(u(2))*cos(u(3))
  Fcn12 : Fcn  Expr=-cos(u(2))*sin(u(3))
  Fcn13 : Fcn  Expr=cos(u(1))*cos(u(3))-sin(u(1))*sin(u(2))*sin(u(3))
  Fcn14 : Fcn  Expr=sin(u(1))*cos(u(3))+cos(u(1))*sin(u(2))*sin(u(3))
  Fcn15 : Fcn  Expr=sin(u(2))
  Fcn16 : Fcn  Expr=-sin(u(1))*cos(u(2))
  Fcn17 : Fcn  Expr=cos(u(1))*cos(u(2))
  Fcn9 : Fcn  Expr=cos(u(2))*cos(u(3))
  Mux1 : Mux  Inputs=9
  RotMat2AxisAngle : Subsystem
  deg2rad : Gain  Gain=pi/180
  xyz 2 zxy : Selector  InputPortWidth=3  IndexOptions=Index vector (dialog)  Indices=[3 1 2]  OutputSizes=1
  zxy 2 xyz : Selector  InputPortWidth=4  IndexOptions=Index vector (dialog)  Indices=[2 3 1 4]  OutputSizes=1
  QuaternionVisu [rad] : Outport
  wires:
  Fcn9/1 -> Mux1/1
  Fcn10/1 -> Mux1/2
  Fcn11/1 -> Mux1/3
  Fcn12/1 -> Mux1/4
  Fcn13/1 -> Mux1/5
  Fcn14/1 -> Mux1/6
  Fcn15/1 -> Mux1/7
  Fcn16/1 -> Mux1/8
  Fcn17/1 -> Mux1/9
  Mux1/1 -> RotMat2AxisAngle/1(RotMat_Visu)  "RotationMatrix Visu"
  RotMat2AxisAngle/1(Angles_Visu) -> zxy 2 xyz/1
  BryantISO [deg]/1 -> xyz 2 zxy/1  "BryantAngles rotx roty rotz Visu"
  deg2rad/1 -> Fcn9/1, Fcn10/1, Fcn11/1, Fcn12/1, Fcn13/1, Fcn14/1, Fcn15/1, Fcn16/1, Fcn17/1
  xyz 2 zxy/1 -> deg2rad/1
  zxy 2 xyz/1 -> QuaternionVisu [rad]/1

== system DvrSimKeybdGD_cs_old/Roewe_550_S_Sedan_1/PreScan_RayCast_Contact_Sensor/Wheels Local to World/conv_RotWheelRL ==
  BryantISO [deg] : Inport
  Fcn10 : Fcn  Expr=cos(u(1))*sin(u(3))+sin(u(1))*sin(u(2))*cos(u(3))
  Fcn11 : Fcn  Expr=sin(u(1))*sin(u(3))-cos(u(1))*sin(u(2))*cos(u(3))
  Fcn12 : Fcn  Expr=-cos(u(2))*sin(u(3))
  Fcn13 : Fcn  Expr=cos(u(1))*cos(u(3))-sin(u(1))*sin(u(2))*sin(u(3))
  Fcn14 : Fcn  Expr=sin(u(1))*cos(u(3))+cos(u(1))*sin(u(2))*sin(u(3))
  Fcn15 : Fcn  Expr=sin(u(2))
  Fcn16 : Fcn  Expr=-sin(u(1))*cos(u(2))
  Fcn17 : Fcn  Expr=cos(u(1))*cos(u(2))
  Fcn9 : Fcn  Expr=cos(u(2))*cos(u(3))
  Mux1 : Mux  Inputs=9
  RotMat2AxisAngle : Subsystem
  deg2rad : Gain  Gain=pi/180
  xyz 2 zxy : Selector  InputPortWidth=3  IndexOptions=Index vector (dialog)  Indices=[3 1 2]  OutputSizes=1
  zxy 2 xyz : Selector  InputPortWidth=4  IndexOptions=Index vector (dialog)  Indices=[2 3 1 4]  OutputSizes=1
  QuaternionVisu [rad] : Outport
  wires:
  Fcn9/1 -> Mux1/1
  Fcn10/1 -> Mux1/2
  Fcn11/1 -> Mux1/3
  Fcn12/1 -> Mux1/4
  Fcn13/1 -> Mux1/5
  Fcn14/1 -> Mux1/6
  Fcn15/1 -> Mux1/7
  Fcn16/1 -> Mux1/8
  Fcn17/1 -> Mux1/9
  Mux1/1 -> RotMat2AxisAngle/1(RotMat_Visu)  "RotationMatrix Visu"
  RotMat2AxisAngle/1(Angles_Visu) -> zxy 2 xyz/1
  BryantISO [deg]/1 -> xyz 2 zxy/1  "BryantAngles rotx roty rotz Visu"
  deg2rad/1 -> Fcn9/1, Fcn10/1, Fcn11/1, Fcn12/1, Fcn13/1, Fcn14/1, Fcn15/1, Fcn16/1, Fcn17/1
  xyz 2 zxy/1 -> deg2rad/1
  zxy 2 xyz/1 -> QuaternionVisu [rad]/1

== system DvrSimKeybdGD_cs_old/Roewe_550_S_Sedan_1/PreScan_RayCast_Contact_Sensor/Wheels Local to World/conv_RotWheelRR ==
  BryantISO [deg] : Inport
  Fcn10 : Fcn  Expr=cos(u(1))*sin(u(3))+sin(u(1))*sin(u(2))*cos(u(3))
  Fcn11 : Fcn  Expr=sin(u(1))*sin(u(3))-cos(u(1))*sin(u(2))*cos(u(3))
  Fcn12 : Fcn  Expr=-cos(u(2))*sin(u(3))
  Fcn13 : Fcn  Expr=cos(u(1))*cos(u(3))-sin(u(1))*sin(u(2))*sin(u(3))
  Fcn14 : Fcn  Expr=sin(u(1))*cos(u(3))+cos(u(1))*sin(u(2))*sin(u(3))
  Fcn15 : Fcn  Expr=sin(u(2))
  Fcn16 : Fcn  Expr=-sin(u(1))*cos(u(2))
  Fcn17 : Fcn  Expr=cos(u(1))*cos(u(2))
  Fcn9 : Fcn  Expr=cos(u(2))*cos(u(3))
  Mux1 : Mux  Inputs=9
  RotMat2AxisAngle : Subsystem
  deg2rad : Gain  Gain=pi/180
  xyz 2 zxy : Selector  InputPortWidth=3  IndexOptions=Index vector (dialog)  Indices=[3 1 2]  OutputSizes=1
  zxy 2 xyz : Selector  InputPortWidth=4  IndexOptions=Index vector (dialog)  Indices=[2 3 1 4]  OutputSizes=1
  QuaternionVisu [rad] : Outport
  wires:
  Fcn9/1 -> Mux1/1
  Fcn10/1 -> Mux1/2
  Fcn11/1 -> Mux1/3
  Fcn12/1 -> Mux1/4
  Fcn13/1 -> Mux1/5
  Fcn14/1 -> Mux1/6
  Fcn15/1 -> Mux1/7
  Fcn16/1 -> Mux1/8
  Fcn17/1 -> Mux1/9
  Mux1/1 -> RotMat2AxisAngle/1(RotMat_Visu)  "RotationMatrix Visu"
  RotMat2AxisAngle/1(Angles_Visu) -> zxy 2 xyz/1
  BryantISO [deg]/1 -> xyz 2 zxy/1  "BryantAngles rotx roty rotz Visu"
  deg2rad/1 -> Fcn9/1, Fcn10/1, Fcn11/1, Fcn12/1, Fcn13/1, Fcn14/1, Fcn15/1, Fcn16/1, Fcn17/1
  xyz 2 zxy/1 -> deg2rad/1
  zxy 2 xyz/1 -> QuaternionVisu [rad]/1

== system DvrSimKeybdGD_cs_old/Roewe_550_S_Sedan_1/PreScan_RayCast_Contact_Sensor/Wheels Local to World/conv_TransWheelFL ==
  transISO [m] : Inport
  Gain1 : Gain  Gain=Gain_xISO
  Gain2 : Gain  Gain=Gain_yISO
  Gain3 : Gain  Gain=Gain_zISO
  Mux2 : Mux  Inputs=3
  Sum : Sum  Inputs=|++
  pos_ini_Visu : Subsystem
  transISO2Visu : Subsystem
  transVisu [m] : Outport
  wires:
  transISO2Visu/3(trans_z_Visu) -> Gain3/1
  transISO2Visu/2(trans_y_Visu) -> Gain2/1
  transISO2Visu/1(trans_x_Visu) -> Gain1/1
  transISO [m]/1 -> transISO2Visu/1(transISO)
  Mux2/1 -> Sum/1
  pos_ini_Visu/1(pos_ini_Visu) -> Sum/2
  Sum/1 -> transVisu [m]/1
  Gain1/1 -> Mux2/1
  Gain2/1 -> Mux2/2
  Gain3/1 -> Mux2/3

== system DvrSimKeybdGD_cs_old/Roewe_550_S_Sedan_1/PreScan_RayCast_Contact_Sensor/Wheels Local to World/conv_TransWheelFR ==
  transISO [m] : Inport
  Gain1 : Gain  Gain=Gain_xISO
  Gain2 : Gain  Gain=Gain_yISO
  Gain3 : Gain  Gain=Gain_zISO
  Mux2 : Mux  Inputs=3
  Sum : Sum  Inputs=|++
  pos_ini_Visu : Subsystem
  transISO2Visu : Subsystem
  transVisu [m] : Outport
  wires:
  transISO2Visu/3(trans_z_Visu) -> Gain3/1
  transISO2Visu/2(trans_y_Visu) -> Gain2/1
  transISO2Visu/1(trans_x_Visu) -> Gain1/1
  transISO [m]/1 -> transISO2Visu/1(transISO)
  Mux2/1 -> Sum/1
  pos_ini_Visu/1(pos_ini_Visu) -> Sum/2
  Sum/1 -> transVisu [m]/1
  Gain1/1 -> Mux2/1
  Gain2/1 -> Mux2/2
  Gain3/1 -> Mux2/3

== system DvrSimKeybdGD_cs_old/Roewe_550_S_Sedan_1/PreScan_RayCast_Contact_Sensor/Wheels Local to World/conv_TransWheelRL ==
  transISO [m] : Inport
  Gain1 : Gain  Gain=Gain_xISO
  Gain2 : Gain  Gain=Gain_yISO
  Gain3 : Gain  Gain=Gain_zISO
  Mux2 : Mux  Inputs=3
  Sum : Sum  Inputs=|++
  pos_ini_Visu : Subsystem
  transISO2Visu : Subsystem
  transVisu [m] : Outport
  wires:
  transISO2Visu/1(trans_x_Visu) -> Gain1/1
  transISO [m]/1 -> transISO2Visu/1(transISO)
  transISO2Visu/2(trans_y_Visu) -> Gain2/1
  transISO2Visu/3(trans_z_Visu) -> Gain3/1
  Mux2/1 -> Sum/1
  pos_ini_Visu/1(pos_ini_Visu) -> Sum/2
  Sum/1 -> transVisu [m]/1
  Gain1/1 -> Mux2/1
  Gain2/1 -> Mux2/2
  Gain3/1 -> Mux2/3
